simulink model "F-LAB6_PART2"  (R2016a)
settings: Solver=VariableStepAuto  StartTime=0.0  StopTime=10.0  RelTol=1e-3
settings Model: Creator=Student  LastModifiedBy=Student

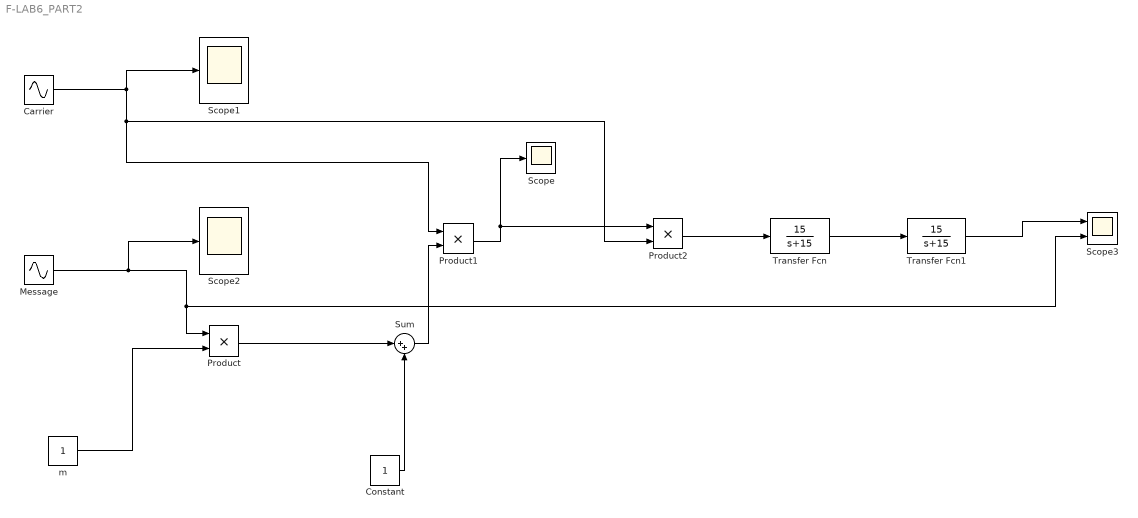
== system F-LAB6_PART2 ==
  " Message" : Sin  Amplitude=2  Frequency=5  SampleTime=0
  Carrier : Sin  Amplitude=2  Frequency=50  SampleTime=0
  Constant : Constant
  Product : Product
  Product1 : Product
  Product2 : Product
  Scope : Scope
  Scope1 : Scope
  Scope2 : Scope
  Scope3 : Scope  NumInputPorts=2
  Sum : Sum  Inputs=|++
  Transfer Fcn : TransferFcn  Numerator=[15]  Denominator=[1 15]
  Transfer Fcn1 : TransferFcn  Numerator=[15]  Denominator=[1 15]
  m : Constant
  wires:
  Carrier/1 -> Product2/2, Product1/1, Scope1/1
  " Message"/1 -> Scope2/1, Product/1, Scope3/2
  m/1 -> Product/2
  Product/1 -> Sum/1
  Constant/1 -> Sum/2
  Sum/1 -> Product1/2
  Product1/1 -> Product2/1, Scope/1
  Product2/1 -> Transfer Fcn/1
  Transfer Fcn/1 -> Transfer Fcn1/1
  Transfer Fcn1/1 -> Scope3/1
